simulink model "Punto3"  (R2017b)
settings: Solver=VariableStepAuto  StartTime=0.0  StopTime=.001  RelTol=1e-3
values from neighbouring files (symbols this model uses):
  dc = [.4 4.2 3]    [Practica5.m]    (also in punto1.m = [.0000001 .0001 1])
  nc = 1    [Practica5.m]    (also in punto1.m)
  p1 = nd(2)*q0    [Practica5.m]    (also in punto1.m)
  p2 = nd(3)*q0    [Practica5.m]    (also in punto1.m)
  q0 = 1/sum(nd)    [Practica5.m]    (also in punto1.m)
  q1 = dd(2)*q0    [Practica5.m]    (also in punto1.m)
  q2 = dd(3)*q0    [Practica5.m]    (also in punto1.m)
  T0 = .5    (= 0.5)    [Practica5.m]    (also in punto1.m = 0.0002)
settings Model: Creator=Agustin  LastModifiedBy=Agustin

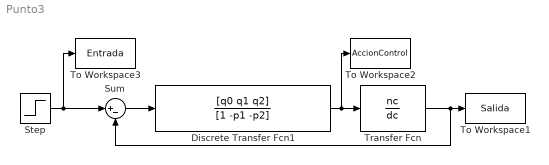
== system Punto3 ==
  Discrete Transfer Fcn1 : DiscreteTransferFcn  Numerator=[q0 q1 q2]  Denominator=[1 -p1 -p2]  SampleTime=T0
  Step : Step  Time=0  After=10  SampleTime=0
  Sum : Sum  Inputs=|+-
  To Workspace1 : ToWorkspace  VariableName=Salida  SaveFormat=Timeseries  SampleTime=-1
  To Workspace2 : ToWorkspace  VariableName=AccionControl  SaveFormat=Timeseries  SampleTime=-1
  To Workspace3 : ToWorkspace  VariableName=Entrada  SaveFormat=Timeseries  SampleTime=-1
  Transfer Fcn : TransferFcn  Numerator=nc  Denominator=dc
  wires:
  Transfer Fcn/1 -> Sum/2, To Workspace1/1
  Sum/1 -> Discrete Transfer Fcn1/1
  Step/1 -> To Workspace3/1, Sum/1
  Discrete Transfer Fcn1/1 -> Transfer Fcn/1, To Workspace2/1
